simulink model "ex_arg_LUT_ref"  (R2024a)
settings: Solver=FixedStepDiscrete  StartTime=0.0  StopTime=10.0  FixedStep=0.2  RelTol=1e-3
model workspace (MAT data in the model file):
  LUT_arg = Simulink.LookupTable
  LUT_arg.Table = Simulink.lookuptable.Table
  LUT_arg.Table.Value = [3  4; 1  2]
  LUT_arg.Table.Dimensions = [2 2]
  LUT_arg.Table.DataType = 'auto'
  LUT_arg.Table.FieldName = 'Table'
  LUT_arg.Breakpoints(1) = Simulink.lookuptable.Breakpoint
  LUT_arg.Breakpoints(1).Value = [1 2]
  LUT_arg.Breakpoints(1).TunableSizeName = 'N1'
  LUT_arg.Breakpoints(1).Dimensions = [1 2]
  LUT_arg.Breakpoints(1).DataType = 'auto'
  LUT_arg.Breakpoints(1).FieldName = 'BP1'
  LUT_arg.Breakpoints(2) = Simulink.lookuptable.Breakpoint
  LUT_arg.Breakpoints(2).Value = [3 4]
  LUT_arg.Breakpoints(2).TunableSizeName = 'N2'
  LUT_arg.Breakpoints(2).Dimensions = [1 2]
  LUT_arg.Breakpoints(2).DataType = 'auto'
  LUT_arg.Breakpoints(2).FieldName = 'BP2'
  LUT_arg.AllowMultipleInstancesOfTypeToHaveDifferentTableBreakpointSizes = 0
  LUT_arg.SupportTunableSize = 0
  LUT_arg.StructTypeInfo = Simulink.lookuptable.StructTypeInfo
  LUT_arg.StructTypeInfo.Name = 'LUT_arg_Type'
  LUT_arg.StructTypeInfo.DataScope = 'Auto'
settings Model: ParameterArgumentNames=LUT_arg  Creator=The MathWorks, Inc.  LastModifiedBy=uditpant
settings SolverCC: AlgebraicLoopSolver=TrustRegion
settings DataIOCC: SaveOutput=off  SignalLogging=off  DSMLogging=off  SaveTime=off  ReturnWorkspaceOutputs=off
settings OptimizationCC: DefaultParameterBehavior=Inlined  EfficientTunableParamExpr=on
settings DebuggingCC: ParameterTunabilityLossMsg=error  UnconnectedInputMsg=warning  UnconnectedOutputMsg=warning  UnconnectedLineMsg=warning  ArithmeticOperatorsInVariantConditions=warning
settings ModelReferenceCC: EnableRefExpFcnMdlSchedulingChecks=on
settings SFSimCC: SimUseLocalCustomCode=off  CustomCodeUndefinedFunction=UseInterfaceOnly
settings RTWCC: Description=Embedded Coder  SystemTargetFile=ert.tlc  TemplateMakefile=ert_default_tmf  GenerateReport=on  RTWVerbose=off  RTWUseLocalCustomCode=off  IncludeHyperlinkInReport=on  LaunchReport=on  GenerateTraceInfo=on  GenerateTraceReport=on  GenerateTraceReportSl=on  GenerateTraceReportSf=on  GenerateTraceReportEml=on  GPUComputeCapability=3.5
settings CodeAppCC: ForceParamTrailComments=on  IgnoreCustomStorageClasses=off  OperatorAnnotations=on  SimulinkDataObjDesc=on  SFDataObjDesc=on  MATLABFcnDesc=on  CustomSymbolStrModelFcn=$N  InsertBlockDesc=on  StateflowObjectComments=on  MATLABSourceComments=on
settings ERTTargetCC: TargetLangStandard=C99 (ISO)  MultiwordLength=2048  GenerateSampleERTMain=on  InlinedParameterPlacement=NonHierarchical  ERTCustomFileTemplate=example_file_process.tlc
settings ConfigComp: CovMetricSettings=dswe

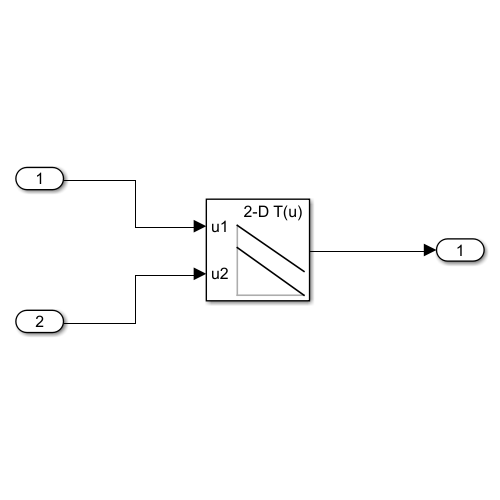
[thumbnail: Simulink's stored preview of the top-level diagram]
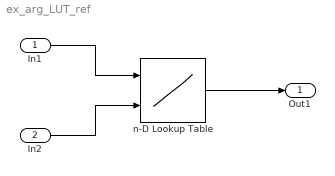
== system ex_arg_LUT_ref ==
  In1 : Inport
  In2 : Inport  Port=2
  n-D Lookup Table : Lookup_n-D  DataSpecification=Lookup table object  LookupTableObject=LUT_arg  BreakpointsForDimension1=[1 2]  BreakpointsForDimension2=[3 4]  BreakpointsForDimension3=[5, 7]  Table=[4 3; 1 2]  InternalRulePriority=Speed  RndMeth=Simplest
      settings: InputPortMap=u0,u1
  Out1 : Outport  VectorParamsAs1DForOutWhenUnconnected=off
  wires:
  In1/1 -> n-D Lookup Table/1
  In2/1 -> n-D Lookup Table/2
  n-D Lookup Table/1 -> Out1/1
